simulink model "updated_simulink_1"  (R2025a)
settings: Solver=VariableStepAuto  StartTime=0.0  StopTime=10  RelTol=1e-3
settings Model: Creator=Aarya  LastModifiedBy=Aarya

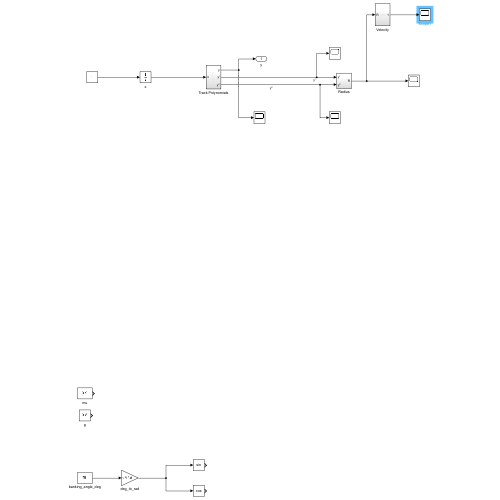
[thumbnail: Simulink's stored preview of the top-level diagram]
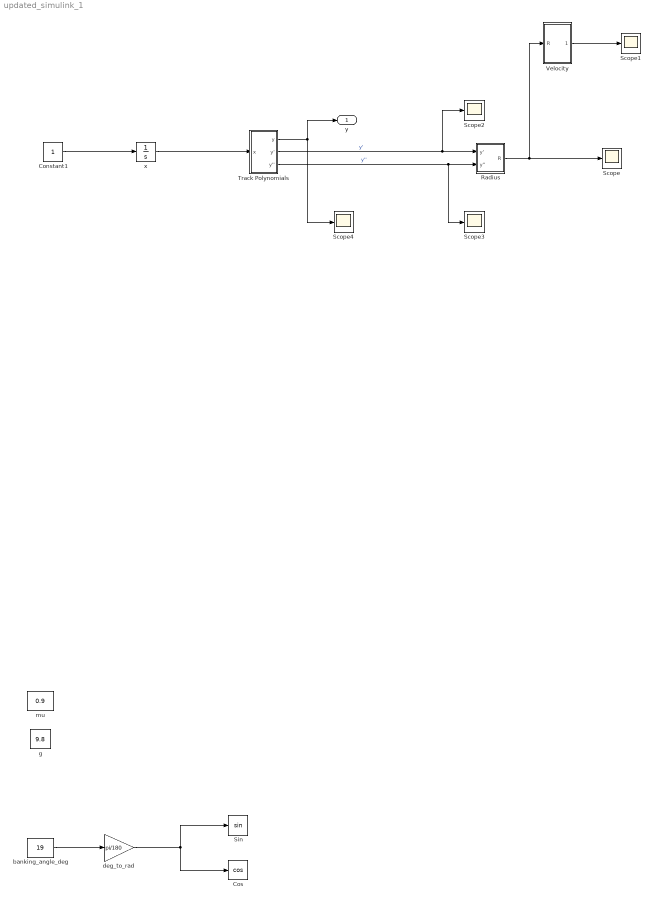
== system updated_simulink_1 ==
  Constant1 : Constant
  Cos : Trigonometry  Operator=cos
  Radius : Subsystem
  Scope{,1..4} (5 alike) : Scope
      Scope settings: ActiveDisplayYMinimum=-6.4833164359872282E+17  ActiveDisplayYMaximum=5.8349847923885066E+18
      Scope1 settings: ActiveDisplayYMinimum=-1.636295819899631E+9  ActiveDisplayYMaximum=1.4726662379514046E+10
      Scope2 settings: ActiveDisplayYMinimum=-220.43999985589514  ActiveDisplayYMaximum=1947.8204444284222  DataLoggingVariableName=ScopeData2
      Scope3 settings: ActiveDisplayYMinimum=-110.37053925258249  ActiveDisplayYMaximum=448.7353983855262  DataLoggingVariableName=ScopeData3
      Scope4 settings: ActiveDisplayYMinimum=-630.54019999999537  ActiveDisplayYMaximum=5745.5897999999543  DataLoggingVariableName=ScopeData4
  Sin : Trigonometry
  Track Polynomials : Subsystem
  Velocity : Subsystem
  banking_angle_deg : Constant  Value=19
  deg_to_rad : Gain  Gain=pi/180
  g : Constant  Value=9.8
  mu : Constant  Value=0.9
  x : Integrator  InitialCondition=6
  y : Outport
  wires:
  banking_angle_deg/1 -> deg_to_rad/1
  deg_to_rad/1 -> Cos/1, Sin/1
  Track Polynomials/1(y) -> Scope4/1, y/1
  Track Polynomials/2(y') -> Scope2/1, Radius/1(y')  "y'"
  Track Polynomials/3(y'') -> Scope3/1, Radius/2(y'')  "y''"
  x/1 -> Track Polynomials/1(x)
  Constant1/1 -> x/1
  Velocity/1(Out1) -> Scope1/1
  Radius/1(R) -> Scope/1, Velocity/1(R)

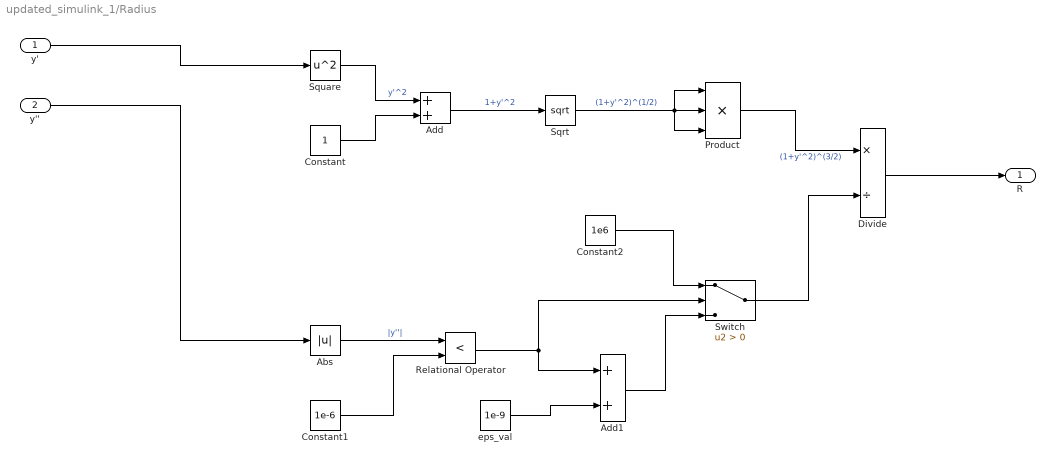
== system updated_simulink_1/Radius ==
  y' : Inport
  y'' : Inport  Port=2
  Abs : Abs  SaturateOnIntegerOverflow=off
  Add : Sum
  Add1 : Sum
  Constant : Constant
  Constant1 : Constant  Value=1e-6
  Constant2 : Constant  Value=1e6
  Divide : Product  Inputs=*/
  Product : Product  Inputs=3
  Relational Operator : RelationalOperator  Operator=<  OutDataTypeStr=boolean  RndMeth=Simplest  InputSameDT=off
  Sqrt : Sqrt
  Square : Math  Operator=square
  Switch : Switch  Criteria=u2 > Threshold  SaturateOnIntegerOverflow=off  InputSameDT=off
  eps_val : Constant  Value=1e-9
  R : Outport
  wires:
  Constant/1 -> Add/2
  Product/1 -> Divide/1  "(1+y'^2)^(3/2)"
  Square/1 -> Add/1  "y'^2"
  Sqrt/1 -> Product/3, Product/1, Product/2  "(1+y'^2)^(1/2)"
  Add/1 -> Sqrt/1  "1+y'^2"
  Divide/1 -> R/1
  eps_val/1 -> Add1/2
  Abs/1 -> Relational Operator/1  "|y''|"
  y'/1 -> Square/1
  y''/1 -> Abs/1
  Constant1/1 -> Relational Operator/2
  Relational Operator/1 -> Switch/2, Add1/1
  Constant2/1 -> Switch/1
  Add1/1 -> Switch/3
  Switch/1 -> Divide/2

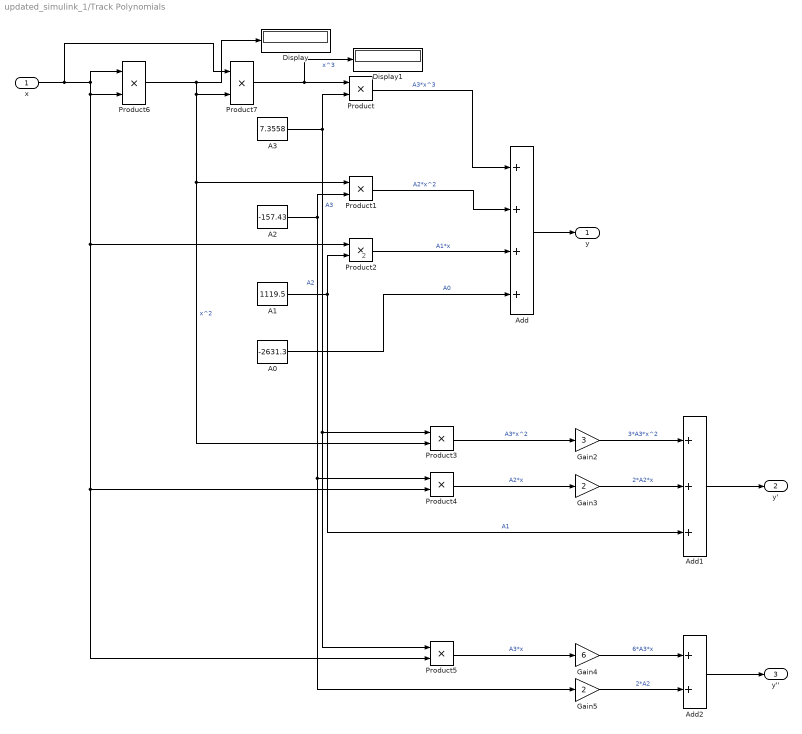
== system updated_simulink_1/Track Polynomials ==
  note: 2
  x : Inport
  A0 : Constant  Value=-2631.3
  A1 : Constant  Value=1119.5
  A2 : Constant  Value=-157.43
  A3 : Constant  Value=7.3558
  Add : Sum  Inputs=++++
  Add1 : Sum  Inputs=+++
  Add2 : Sum
  Display : Display
  Display1 : Display
  Gain2 : Gain  Gain=3
  Gain3 : Gain  Gain=2
  Gain4 : Gain  Gain=6
  Gain5 : Gain  Gain=2
  Product{,1..7} (8 alike) : Product
  y : Outport
  y' : Outport  Port=2
  y'' : Outport  Port=3
  wires:
  A3/1 -> Product5/1, Product3/1, Product/2  "A3"
  A1/1 -> Add1/3, Product2/2  "A1"
  x/1 -> Product7/1, Product5/2, Product4/2, Product2/1, Product6/2, Product6/1
  Product6/1 -> Display/1, Product7/2, Product3/2, Product1/1  "x^2"
  Add/1 -> y/1
  Gain3/1 -> Add1/2  "2*A2*x"
  A2/1 -> Gain5/1, Product4/1, Product1/2  "A2"
  Add2/1 -> y''/1
  Product1/1 -> Add/2  "A2*x^2"
  Add1/1 -> y'/1
  A0/1 -> Add/4  "A0"
  Product2/1 -> Add/3  "A1*x"
  Product/1 -> Add/1  "A3*x^3"
  Gain4/1 -> Add2/1  "6*A3*x"
  Product4/1 -> Gain3/1  "A2*x"
  Product7/1 -> Display1/1, Product/1  "x^3"
  Product5/1 -> Gain4/1  "A3*x"
  Product3/1 -> Gain2/1  "A3*x^2"
  Gain5/1 -> Add2/2  "2*A2"
  Gain2/1 -> Add1/1  "3*A3*x^2"

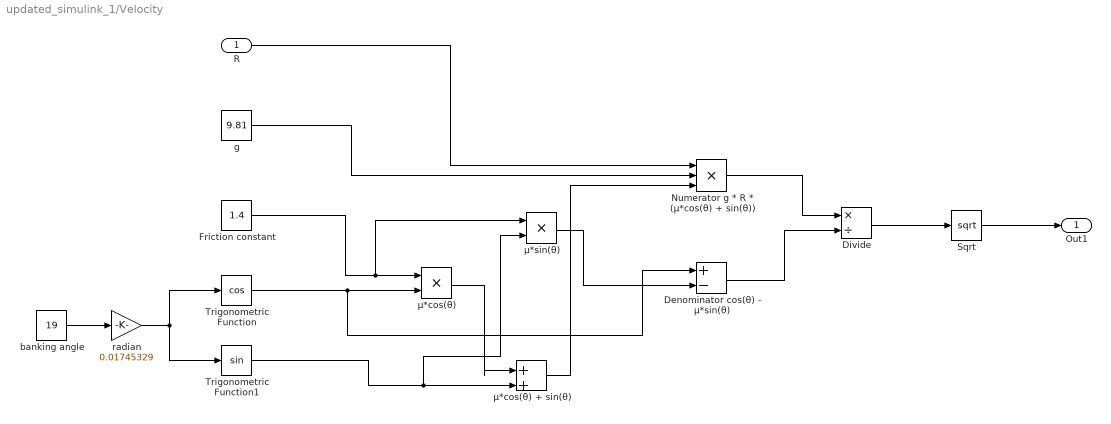
== system updated_simulink_1/Velocity ==
  R : Inport
  Denominator cos(θ) - μ*sin(θ) : Sum  Inputs=+-
  Divide : Product  Inputs=*/
  Friction constant : Constant  Value=1.4
  Numerator g * R * (μ*cos(θ) + sin(θ)) : Product  Inputs=3
  Sqrt : Sqrt
  Trigonometric Function : Trigonometry  Operator=cos
  Trigonometric Function1 : Trigonometry
  banking angle : Constant  Value=19
  g : Constant  Value=9.81
  radian : Gain  Gain=0.01745329
  μ*cos(θ) : Product
  μ*cos(θ) + sin(θ) : Sum  Inputs=|++
  μ*sin(θ) : Product
  Out1 : Outport
  wires:
  radian/1 -> Trigonometric Function/1, Trigonometric Function1/1
  banking angle/1 -> radian/1
  Trigonometric Function/1 -> Denominator cos(θ) - μ*sin(θ)/1, μ*cos(θ)/2
  Friction constant/1 -> μ*sin(θ)/1, μ*cos(θ)/1
  μ*cos(θ)/1 -> μ*cos(θ) + sin(θ)/1
  Trigonometric Function1/1 -> μ*sin(θ)/2, μ*cos(θ) + sin(θ)/2
  R/1 -> Numerator g * R * (μ*cos(θ) + sin(θ))/1
  g/1 -> Numerator g * R * (μ*cos(θ) + sin(θ))/2
  μ*cos(θ) + sin(θ)/1 -> Numerator g * R * (μ*cos(θ) + sin(θ))/3
  μ*sin(θ)/1 -> Denominator cos(θ) - μ*sin(θ)/2
  Numerator g * R * (μ*cos(θ) + sin(θ))/1 -> Divide/1
  Denominator cos(θ) - μ*sin(θ)/1 -> Divide/2
  Divide/1 -> Sqrt/1
  Sqrt/1 -> Out1/1
